simulink model "battery_few_sim"  (R2022a)
settings: Solver=VariableStepAuto  StartTime=0.0  StopTime=1500  RelTol=1e-3
undefined symbols (not defined in the file): R_AIR, T_AMB
libraries: fl_lib x9, ee_lib x6, nesl_utility x4
settings Model: DataDictionary=battery.sldd  Creator=Cristobal  LastModifiedBy=Cristobal
settings SFSimCC: SimTargetLang=C++  GPUAcceleration=on  SimDLTargetLibrary=cudnn

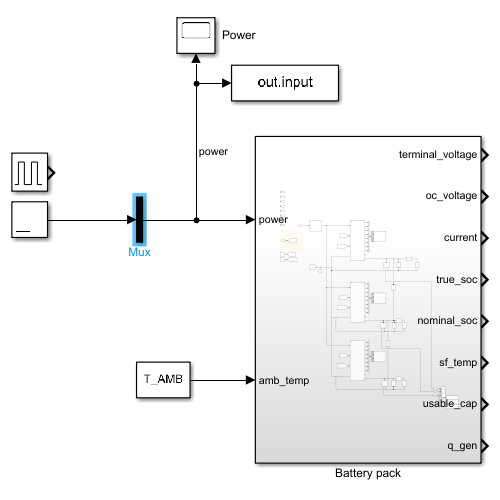
[thumbnail: Simulink's stored preview of the top-level diagram]
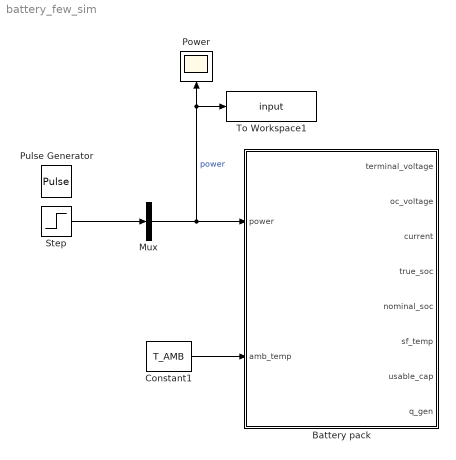
== system battery_few_sim ==
  Battery pack : Subsystem
  Constant1 : Constant  Value=T_AMB
  Mux : Mux  Inputs=1
  Power : Scope
  Pulse Generator : DiscretePulseGenerator  PulseType=Time based  Amplitude=1e-1  Period=300  PulseWidth=50
  Step : Step  Time=0  After=80  SampleTime=0
  To Workspace1 : ToWorkspace  VariableName=input  SaveFormat=Timeseries  SampleTime=-1
  wires:
  Constant1/1 -> Battery pack/2(amb_temp)
  Mux/1 -> To Workspace1/1, Power/1, Battery pack/1(power)  "power"
  Step/1 -> Mux/1

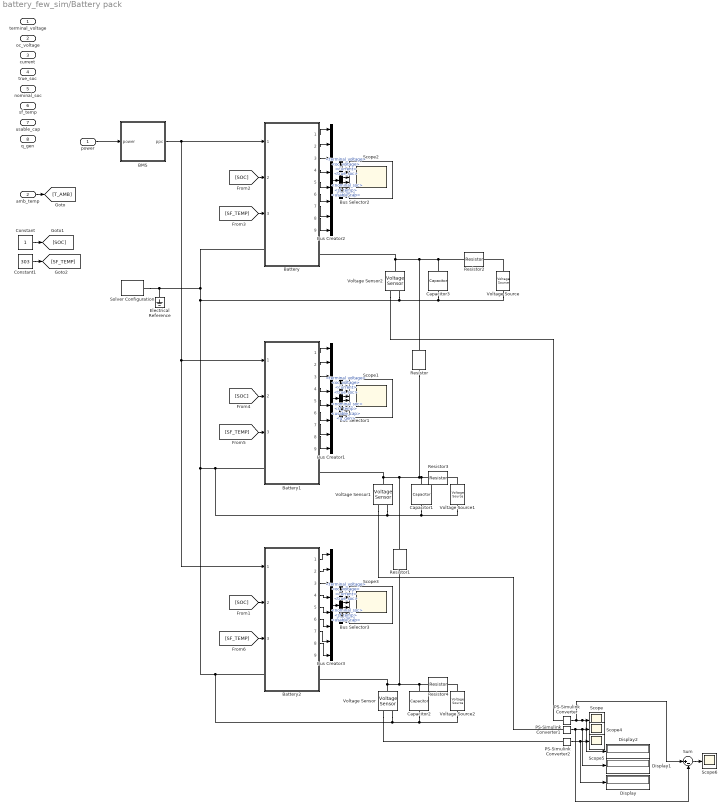
== system battery_few_sim/Battery pack ==
  power : Inport
  amb_temp : Inport  Port=2
  BMS : Subsystem  mask{Outputs=3}
      mask init:
      | % for i = 1:Outputs
      |     %     replace_block(gcb, "Name", "Terminator" + i, "Outport", "noprompt");
      |     % end
      |     % for i = Outputs + 1:64
      |     %     replace_block(gcb, "Name", "Terminator" + i, "Terminator", "noprompt");
      |     % end
      mask DialogControl DescGroupVar Prompt: BMS
      mask DialogControl DescTextVar Prompt: Ideal BMS that evenly distributes power
  Battery : Subsystem  ReferencedSubsystem=battery
  Battery1 : Subsystem  ReferencedSubsystem=battery
  Battery2 : Subsystem  ReferencedSubsystem=battery
  Bus Creator1 : BusCreator  Inputs=8
  Bus Creator2 : BusCreator  Inputs=8
  Bus Creator3 : BusCreator  Inputs=8
  Bus Selector1 : BusSelector  OutputSignals=terminal_voltage,oc_voltage,current,true_soc,nominal_soc,sf_temp,usable_cap,q_gen
  Bus Selector2 : BusSelector  OutputSignals=terminal_voltage,oc_voltage,current,true_soc,nominal_soc,sf_temp,usable_cap,q_gen
  Bus Selector3 : BusSelector  OutputSignals=terminal_voltage,oc_voltage,current,true_soc,nominal_soc,sf_temp,usable_cap,q_gen
  Capacitor1 : ee_lib/Passive/Capacitor  cap_option=0  c=C_AIR F  Cvec=[1e-05, 1e-06] F  Vvec=[0, 10] V  CV_table_symmetry=1  f_vec=[1, 10] kHz  DFext_vec=[.8, 1.2]  enable_C_tol=0  C_tol=5  tol_distribution=1  nSigma=4  r=0 Ohm  g=0 1/Ohm  averaging_period=0 s  enable_operating_limits=0  operating_limit_action=2  max_working_voltage_range=[-25, 25] V  power_rating=1 W  enable_faults=0  fault_action=1  Cscale_faulted=100  R_faulted=1e-3 Ohm  G_faulted=0 1/Ohm  tau_fault=1e-3 s  enable_temporal_fault=0  t_fault=1 s  enable_behavioral_fault=0  max_permissible_voltage_range=[-100, 100] V  t_fail_on_voltage=1 s  i_specify=off  i_priority=None  i=0 A  i_nominal_specify=off  i_nominal_unit=A  i_nominal_value=1  v_specify=off  v_priority=None  v=0 V  v_nominal_specify=off  v_nominal_unit=V  v_nominal_value=1  vc_specify=on  vc_priority=High  vc=T_AMB V  vc_nominal_specify=off  vc_nominal_unit=V  vc_nominal_value=1
  Capacitor2 : ee_lib/Passive/Capacitor  cap_option=0  c=C_AIR F  Cvec=[1e-05, 1e-06] F  Vvec=[0, 10] V  CV_table_symmetry=1  f_vec=[1, 10] kHz  DFext_vec=[.8, 1.2]  enable_C_tol=0  C_tol=5  tol_distribution=1  nSigma=4  r=0 Ohm  g=0 1/Ohm  averaging_period=0 s  enable_operating_limits=0  operating_limit_action=2  max_working_voltage_range=[-25, 25] V  power_rating=1 W  enable_faults=0  fault_action=1  Cscale_faulted=100  R_faulted=1e-3 Ohm  G_faulted=0 1/Ohm  tau_fault=1e-3 s  enable_temporal_fault=0  t_fault=1 s  enable_behavioral_fault=0  max_permissible_voltage_range=[-100, 100] V  t_fail_on_voltage=1 s  i_specify=off  i_priority=None  i=0 A  i_nominal_specify=off  i_nominal_unit=A  i_nominal_value=1  v_specify=off  v_priority=None  v=0 V  v_nominal_specify=off  v_nominal_unit=V  v_nominal_value=1  vc_specify=on  vc_priority=High  vc=T_AMB V  vc_nominal_specify=off  vc_nominal_unit=V  vc_nominal_value=1
  Capacitor3 : ee_lib/Passive/Capacitor  cap_option=0  c=C_AIR F  Cvec=[1e-05, 1e-06] F  Vvec=[0, 10] V  CV_table_symmetry=1  f_vec=[1, 10] kHz  DFext_vec=[.8, 1.2]  enable_C_tol=0  C_tol=5  tol_distribution=1  nSigma=4  r=0 Ohm  g=0 1/Ohm  averaging_period=0 s  enable_operating_limits=0  operating_limit_action=2  max_working_voltage_range=[-25, 25] V  power_rating=1 W  enable_faults=0  fault_action=1  Cscale_faulted=100  R_faulted=1e-3 Ohm  G_faulted=0 1/Ohm  tau_fault=1e-3 s  enable_temporal_fault=0  t_fault=1 s  enable_behavioral_fault=0  max_permissible_voltage_range=[-100, 100] V  t_fail_on_voltage=1 s  i_specify=off  i_priority=None  i=0 A  i_nominal_specify=off  i_nominal_unit=A  i_nominal_value=1  v_specify=off  v_priority=None  v=0 V  v_nominal_specify=off  v_nominal_unit=V  v_nominal_value=1  vc_specify=on  vc_priority=High  vc=T_AMB V  vc_nominal_specify=off  vc_nominal_unit=V  vc_nominal_value=1
  Constant : Constant
  Constant1 : Constant  Value=303
  Display : Display
  Display1 : Display
  Display2 : Display
  Electrical Reference : fl_lib/Electrical/Electrical Elements/Electrical Reference
      settings: SourceProductBaseCode=PW,SS,VE
  PS-Simulink Converter : nesl_utility/PS-Simulink Converter  PhysicalDomain=network_engine_domain  SubClassName=ps_output  LeftPortType=input  RightPortType=output  PseudoPeriodic=off  Frequencies=[]  VectorFormat=inherit  Unit=inherit  AffineConversion=off
      settings: SourceProductBaseCode=SS,PW,VE
  PS-Simulink Converter1 : nesl_utility/PS-Simulink Converter  PhysicalDomain=network_engine_domain  SubClassName=ps_output  LeftPortType=input  RightPortType=output  PseudoPeriodic=off  Frequencies=[]  VectorFormat=inherit  Unit=inherit  AffineConversion=off
      settings: SourceProductBaseCode=SS,PW,VE
  PS-Simulink Converter2 : nesl_utility/PS-Simulink Converter  PhysicalDomain=network_engine_domain  SubClassName=ps_output  LeftPortType=input  RightPortType=output  PseudoPeriodic=off  Frequencies=[]  VectorFormat=inherit  Unit=inherit  AffineConversion=off
      settings: SourceProductBaseCode=SS,PW,VE
  Resistor : fl_lib/Electrical/Electrical Elements/Resistor  R=1e3 Ohm  i_specify=off  i_priority=None  i=0 A  i_nominal_specify=off  i_nominal_unit=A  i_nominal_value=1  v_specify=off  v_priority=None  v=0 V  v_nominal_specify=off  v_nominal_unit=V  v_nominal_value=1
      settings: SourceProductBaseCode=PW,SS,VE
  Resistor1 : fl_lib/Electrical/Electrical Elements/Resistor  R=1e3 Ohm  i_specify=off  i_priority=None  i=0 A  i_nominal_specify=off  i_nominal_unit=A  i_nominal_value=1  v_specify=off  v_priority=None  v=0 V  v_nominal_specify=off  v_nominal_unit=V  v_nominal_value=1
      settings: SourceProductBaseCode=PW,SS,VE
  Resistor2 : fl_lib/Electrical/Electrical Elements/Resistor  R=R_AIR Ohm  i_specify=off  i_priority=None  i=0 A  i_nominal_specify=off  i_nominal_unit=A  i_nominal_value=1  v_specify=off  v_priority=None  v=0 V  v_nominal_specify=off  v_nominal_unit=V  v_nominal_value=1
      settings: SourceProductBaseCode=PW,SS,VE
  Resistor3 : fl_lib/Electrical/Electrical Elements/Resistor  R=1e12 Ohm  i_specify=off  i_priority=None  i=0 A  i_nominal_specify=off  i_nominal_unit=A  i_nominal_value=1  v_specify=off  v_priority=None  v=0 V  v_nominal_specify=off  v_nominal_unit=V  v_nominal_value=1
      settings: SourceProductBaseCode=PW,SS,VE
  Resistor4 : fl_lib/Electrical/Electrical Elements/Resistor  R=R_AIR Ohm  i_specify=off  i_priority=None  i=0 A  i_nominal_specify=off  i_nominal_unit=A  i_nominal_value=1  v_specify=off  v_priority=None  v=0 V  v_nominal_specify=off  v_nominal_unit=V  v_nominal_value=1
      settings: SourceProductBaseCode=PW,SS,VE
  Scope{,4..6} (4 alike) : Scope
  Scope1 : Scope  NumInputPorts=8
  Scope2 : Scope  NumInputPorts=8
  Scope3 : Scope  NumInputPorts=8
  Solver Configuration : nesl_utility/Solver Configuration  PhysicalDomain=network_engine_domain  SubClassName=solver  LeftPortType=input  RightPortType=generic  Tones=[]  Harmonics=[]  SimulateNoise=off  Profile=off  UseLocalSampling=off  EnableSwitchedLinearOptims=on  FrequencyDomain=off  UseCCode=off  RelTol=0.001  AbsTol=0.001  MinStep=1e-09  ToWorkspace=off  RevertToSquareIcSolve=off  NumHomotopyIterations=100  PhasorMode=off  PhasorModeNumHarmonics=1  IndexReductionMethod=DerivativeReplacement  DoDC=off  ResidualTolerance=1e-09  UseLocalSolver=off  LocalSolverChoice=NE_BACKWARD_EULER_ADVANCER  LocalSolverSampleTime=0.001  DoFixedCost=off  MaxNonlinIter=3  MaxModeIter=2  ComputeImpulses=off  ImpulseIterations=2  LinearAlgebra=auto  LinearAlgebraNumThread=0  EquationFormulation=NE_TIME_EF  DelaysMemoryBudget=1024  AutomaticFiltering=on  FilteringTimeConstant=0.001  PartitionStorageMethod=AS_NEEDED  PartitionMemoryBudget=1024  PartitionMethod=ROBUST
      settings: SourceProductBaseCode=SS,PW,VE
  Sum : Sum  Inputs=|+-
  Voltage Sensor : fl_lib/Electrical/Electrical Sensors/Voltage Sensor
      settings: SourceProductBaseCode=PW,SS,VE
  Voltage Sensor1 : fl_lib/Electrical/Electrical Sensors/Voltage Sensor
      settings: SourceProductBaseCode=PW,SS,VE
  Voltage Sensor2 : fl_lib/Electrical/Electrical Sensors/Voltage Sensor
      settings: SourceProductBaseCode=PW,SS,VE
  Voltage Source : ee_lib/Sources/Voltage Source  dc_voltage=T_AMB V  ac_voltage=0 V  ac_shift=0 rad  ac_frequency=60 Hz  noise_mode=0  PSD=0 V^2/Hz  repeatability=1  auto_seed=3499211588  user_seed=0  sample_time=1e-3 s  i_specify=off  i_priority=None  i=0 A  i_nominal_specify=off  i_nominal_unit=A  i_nominal_value=1  v_specify=off  v_priority=None  v=0 V  v_nominal_specify=off  v_nominal_unit=V  v_nominal_value=1
  Voltage Source1 : ee_lib/Sources/Voltage Source  dc_voltage=T_AMB V  ac_voltage=0 V  ac_shift=0 rad  ac_frequency=60 Hz  noise_mode=0  PSD=0 V^2/Hz  repeatability=1  auto_seed=3890346746  user_seed=0  sample_time=1e-3 s  i_specify=off  i_priority=None  i=0 A  i_nominal_specify=off  i_nominal_unit=A  i_nominal_value=1  v_specify=off  v_priority=None  v=0 V  v_nominal_specify=off  v_nominal_unit=V  v_nominal_value=1
  Voltage Source2 : ee_lib/Sources/Voltage Source  dc_voltage=T_AMB V  ac_voltage=0 V  ac_shift=0 rad  ac_frequency=60 Hz  noise_mode=0  PSD=0 V^2/Hz  repeatability=1  auto_seed=3922919431  user_seed=0  sample_time=1e-3 s  i_specify=off  i_priority=None  i=0 A  i_nominal_specify=off  i_nominal_unit=A  i_nominal_value=1  v_specify=off  v_priority=None  v=0 V  v_nominal_specify=off  v_nominal_unit=V  v_nominal_value=1
  terminal_voltage : Outport
  oc_voltage : Outport  Port=2
  current : Outport  Port=3
  true_soc : Outport  Port=4
  nominal_soc : Outport  Port=5
  sf_temp : Outport  Port=6
  usable_cap : Outport  Port=7
  q_gen : Outport  Port=8
  wires:
  Bus Selector1/1 -> Scope1/1  "<terminal_voltage>"
  Bus Selector1/6 -> Scope1/6  "<sf_temp>"
  Bus Selector1/7 -> Scope1/7  "<usable_cap>"
  Bus Selector1/3 -> Scope1/3  "<current>"
  Bus Selector1/5 -> Scope1/5  "<nominal_soc>"
  Bus Selector1/2 -> Scope1/2  "<oc_voltage>"
  Bus Selector1/4 -> Scope1/4  "<true_soc>"
  Bus Selector1/8 -> Scope1/8  "<q_gen>"
  Battery1/1 -> Bus Creator1/1
  Battery1/2 -> Bus Creator1/2
  Battery1/3 -> Bus Creator1/3
  Battery1/4 -> Bus Creator1/4
  Battery1/5 -> Bus Creator1/5
  Battery1/6 -> Bus Creator1/6
  Battery1/7 -> Bus Creator1/7
  Battery1/8 -> Bus Creator1/8
  Bus Creator1/1 -> Bus Selector1/1
  amb_temp/1 -> [T_AMB]
  [SF_TEMP] -> Battery/3
  Constant/1 -> [SOC]
  Constant1/1 -> [SF_TEMP]
  [SOC] -> Battery/2
  [SOC] -> Battery1/2
  power/1 -> BMS/1(power)
  BMS/1(ppc) -> Battery2/1, Battery1/1, Battery/1
  Bus Creator2/1 -> Bus Selector2/1
  Bus Selector2/8 -> Scope2/8  "<q_gen>"
  Bus Selector2/4 -> Scope2/4  "<true_soc>"
  Bus Selector2/2 -> Scope2/2  "<oc_voltage>"
  Bus Selector2/5 -> Scope2/5  "<nominal_soc>"
  Bus Selector2/3 -> Scope2/3  "<current>"
  Bus Selector2/7 -> Scope2/7  "<usable_cap>"
  Bus Selector2/6 -> Scope2/6  "<sf_temp>"
  Bus Selector2/1 -> Scope2/1  "<terminal_voltage>"
  Battery/1 -> Bus Creator2/1
  Battery/2 -> Bus Creator2/2
  Battery/3 -> Bus Creator2/3
  Battery/4 -> Bus Creator2/4
  Battery/5 -> Bus Creator2/5
  Battery/6 -> Bus Creator2/6
  Battery/7 -> Bus Creator2/7
  Battery/8 -> Bus Creator2/8
  [SF_TEMP] -> Battery1/3
  [SF_TEMP] -> Battery2/3
  [SOC] -> Battery2/2
  Bus Creator3/1 -> Bus Selector3/1
  Battery2/8 -> Bus Creator3/8
  Battery2/7 -> Bus Creator3/7
  Battery2/6 -> Bus Creator3/6
  Battery2/5 -> Bus Creator3/5
  Battery2/4 -> Bus Creator3/4
  Bus Selector3/8 -> Scope3/8  "<q_gen>"
  Bus Selector3/4 -> Scope3/4  "<true_soc>"
  Bus Selector3/2 -> Scope3/2  "<oc_voltage>"
  Bus Selector3/5 -> Scope3/5  "<nominal_soc>"
  Bus Selector3/3 -> Scope3/3  "<current>"
  Bus Selector3/7 -> Scope3/7  "<usable_cap>"
  Bus Selector3/6 -> Scope3/6  "<sf_temp>"
  Bus Selector3/1 -> Scope3/1  "<terminal_voltage>"
  Battery2/3 -> Bus Creator3/3
  Battery2/2 -> Bus Creator3/2
  Battery2/1 -> Bus Creator3/1
  PS-Simulink Converter/1 -> Sum/1, Display2/1, Scope/1
  PS-Simulink Converter1/1 -> Sum/2, Display1/1, Scope4/1
  PS-Simulink Converter2/1 -> Display/1, Scope5/1
  Sum/1 -> Scope6/1
  connections:
  Voltage Source2/RConn1 -- Capacitor2/RConn1 -- Voltage Sensor/RConn2 -- Voltage Sensor2/RConn2 -- Capacitor3/RConn1 -- Voltage Source/RConn1 -- Electrical Reference/LConn1 -- Solver Configuration/RConn1 -- Battery/LConn1 -- Capacitor1/RConn1 -- Voltage Source1/RConn1 -- Voltage Sensor1/RConn2 -- Battery1/LConn1 -- Battery2/LConn1
  Voltage Sensor2/LConn1 -- Battery/RConn2 -- Resistor2/LConn1 -- Capacitor3/LConn1 -- Resistor/LConn1
  Resistor/RConn1 -- Resistor3/LConn1 -- Capacitor1/LConn1 -- Resistor1/LConn1 -- Battery1/RConn2 -- Voltage Sensor1/LConn1
  Capacitor2/LConn1 -- Resistor1/RConn1 -- Battery2/RConn2 -- Voltage Sensor/LConn1 -- Resistor4/LConn1
  Voltage Sensor/RConn1 -- PS-Simulink Converter2/LConn1
  Voltage Sensor1/RConn1 -- PS-Simulink Converter1/LConn1
  Voltage Sensor2/RConn1 -- PS-Simulink Converter/LConn1
  Voltage Source/LConn1 -- Resistor2/RConn1
  Voltage Source1/LConn1 -- Resistor3/RConn1
  Voltage Source2/LConn1 -- Resistor4/RConn1

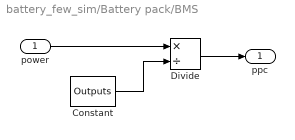
== system battery_few_sim/Battery pack/BMS ==
  power : Inport
  Constant : Constant  Value=Outputs
  Divide : Product  Inputs=*/
  ppc : Outport
  wires:
  Constant/1 -> Divide/2
  power/1 -> Divide/1
  Divide/1 -> ppc/1
